simulink model "HW9_P6_tmrpns_2"  (R2015b)
settings: Solver=ode3  StartTime=0.0  StopTime=40  FixedStep=0.001  RelTol=1e-3
values from neighbouring files (symbols this model uses):
  F = [-2-wn^2  -3-wn^2-2*ze*wn]    [HW9_P6_1.m]
  x10 = 2    [HW9_P6_1.m]
  x20 = 0    [HW9_P6_1.m]
settings Model: ExtModeTrigMode=oneshot  ExtModeArmWhenConnect=off  Creator=BC  LastModifiedBy=bcc88
settings DataIOCC: LimitDataPoints=off  SaveFormat=Array  SignalLoggingSaveFormat=ModelDataLogs
settings OptimizationCC: BlockReduction=off  BooleanDataType=off  ExpressionDepthLimit=2147483647  InitFltsAndDblsToZero=on
settings DebuggingCC: SaveWithParameterizedLinksMsg=none  UnderspecifiedInitializationDetection=Classic  MergeDetectMultiDrivingBlocksExec=none  SignalResolutionControl=TryResolveAllWithWarning  MultiTaskDSMMsg=warning  MultiTaskCondExecSysMsg=none  FcnCallInpInsideContextMsg=UseLocalSettings  StateNameClashWarn=warning
settings HardwareCC: ProdBitPerPointer=32  ProdLargestAtomicFloat=None  ProdIntDivRoundTo=Undefined  ProdEndianess=Unspecified  ProdWordSize=32  ProdHWDeviceType=32-bit Generic  TargetUnknown=on
settings GRTTargetCC: TargetFcnLib=ansi_tfl_tmw.mat  CombineOutputUpdateFcns=off  GRTInterface=on
settings ConfigComp: CovModelRefEnable=Off

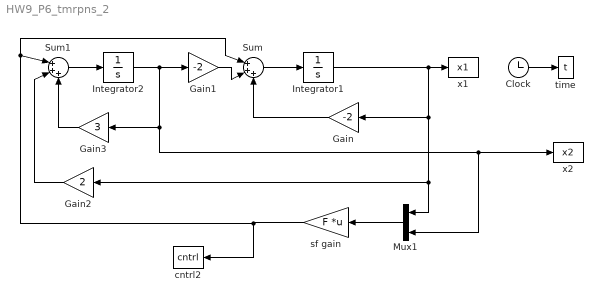
== system HW9_P6_tmrpns_2 ==
  Clock : Clock
  Gain : Gain  Gain=-2
  Gain1 : Gain  Gain=-2
  Gain2 : Gain  Gain=2
  Gain3 : Gain  Gain=3
  Integrator1 : Integrator  InitialCondition=x10
  Integrator2 : Integrator  InitialCondition=x20
  Mux1 : Mux  Inputs=2
  Sum : Sum  Inputs=|+++
  Sum1 : Sum  Inputs=|+++
  cntrl2 : ToWorkspace  VariableName=cntrl  SampleTime=-1
  sf gain : Gain  Gain=F  Multiplication=Matrix(K*u)
  time : ToWorkspace  VariableName=t  SampleTime=-1
  x1 : ToWorkspace  VariableName=x1  SampleTime=-1
  x2 : ToWorkspace  VariableName=x2  SampleTime=-1
  wires:
  Clock/1 -> time/1
  Mux1/1 -> sf gain/1
  sf gain/1 -> Sum/1, Sum1/1, cntrl2/1
  Integrator1/1 -> x1/1, Gain/1, Mux1/1, Gain2/1
  Sum/1 -> Integrator1/1
  Integrator2/1 -> Gain1/1, Gain3/1, Mux1/2, x2/1
  Sum1/1 -> Integrator2/1
  Gain1/1 -> Sum/2
  Gain/1 -> Sum/3
  Gain3/1 -> Sum1/3
  Gain2/1 -> Sum1/2
